simulink model "adarbha_HW9_sim_take2"  (Simulink 7.7)
settings: Solver=ode45  StartTime=0.0  StopTime=10.0  RelTol=1e-3
undefined symbols (not defined in the file): Area, Cd, density, Time, time_s, vel_m_s, Velocity_kph, weight_N
libraries: simulink x1
settings Model: Creator=Arjun  LastModifiedBy=Arjun

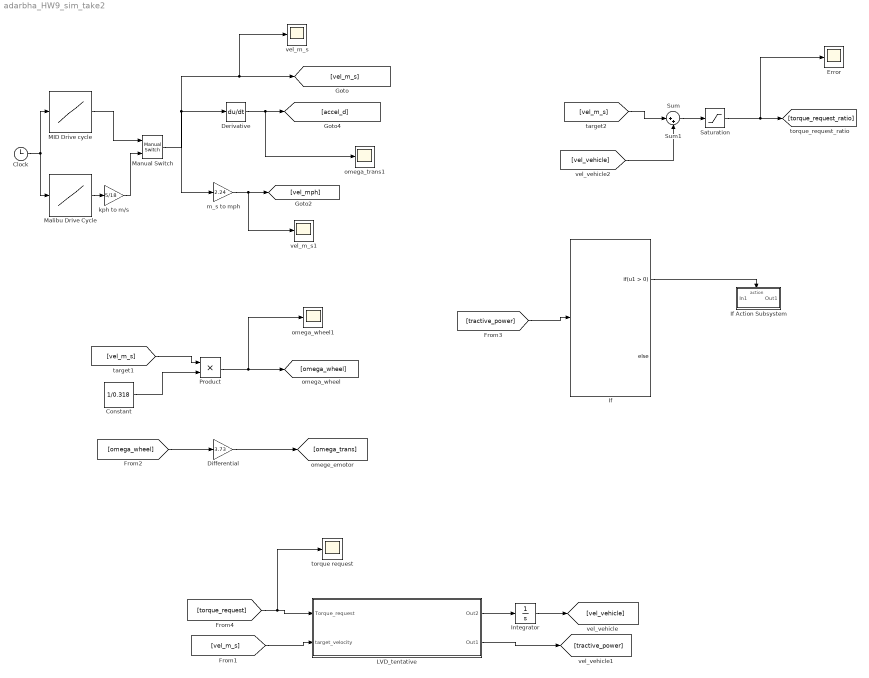
== system adarbha_HW9_sim_take2 ==
  Clock : Clock
      settings: Decimation=10
  Constant : Constant  Value=1/0.318
  Derivative : Derivative
  Differential : Gain  Gain=3.73
  Error : Scope
      settings: SaveName=ScopeData11
  If : If
  If Action Subsystem : Subsystem  TreatAsAtomicUnit=on
  Integrator : Integrator
  LVD_tentative : Subsystem
  MID Drive cycle : Lookup_n-D  NumberOfTableDimensions=1  BreakpointsForDimension1=time_s  Table=vel_m_s  RndMeth=Simplest  InputSameDT=on
  Malibu Drive Cycle : Lookup_n-D  NumberOfTableDimensions=1  BreakpointsForDimension1=Time  Table=Velocity_kph  RndMeth=Simplest  InputSameDT=on
  Manual Switch : simulink/Signal Routing/Manual Switch  SystemSampleTime=-1  sw=0  action=0  varsize=off
  Product : Product  RndMeth=Zero
  Saturation : Saturate  UpperLimit=1  LowerLimit=-1
  Sum : Sum  Inputs=|+-
  Sum1 : Sum  Inputs=|++
  kph to m/s : Gain  Gain=5/18
  m_s to mph : Gain  Gain=2.24
  omega_trans1 : Scope
      settings: YMin=0  YMax=40
  omega_wheel1 : Scope
      settings: SaveName=ScopeData3
  torque request : Scope
      settings: SaveName=ScopeData4
  vel_m_s : Scope
      settings: TimeRange=49.80784012298233  YMin=0  YMax=30
  vel_m_s1 : Scope
      settings: YMin=0  YMax=40  SaveName=ScopeData2
  wires:
  m_s to mph/1 -> [vel_mph], vel_m_s1/1
  Clock/1 -> MID Drive cycle/1, Malibu Drive Cycle/1
  MID Drive cycle/1 -> Manual Switch/1
  Manual Switch/1 -> m_s to mph/1, [vel_m_s], vel_m_s/1, Derivative/1
  Malibu Drive Cycle/1 -> kph to m/s/1
  kph to m/s/1 -> Manual Switch/2
  Derivative/1 -> [accel_d], omega_trans1/1
  [vel_m_s] -> Product/1
  Product/1 -> [omega_wheel], omega_wheel1/1
  Constant/1 -> Product/2
  [omega_wheel] -> Differential/1
  Differential/1 -> [omega_trans]
  [vel_m_s] -> LVD_tentative/2(target_velocity)
  [torque_request] -> LVD_tentative/1(Torque_request), torque request/1
  Integrator/1 -> [vel_vehicle]
  LVD_tentative/1(Out2) -> Integrator/1
  [vel_m_s] -> Sum/1
  [vel_vehicle] -> Sum/2
  Sum/1 -> Saturation/1
  Saturation/1 -> Error/1, [torque_request_ratio]
  LVD_tentative/2(Out1) -> [tractive_power]
  [tractive_power] -> If/1
  If/1 -> If Action Subsystem/Action

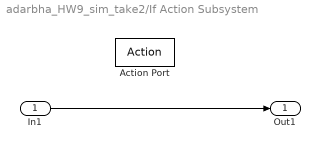
== system adarbha_HW9_sim_take2/If Action Subsystem ==
  In1 : Inport
  Action Port : ActionPort  ActionType=then
  Out1 : Outport
  wires:
  In1/1 -> Out1/1

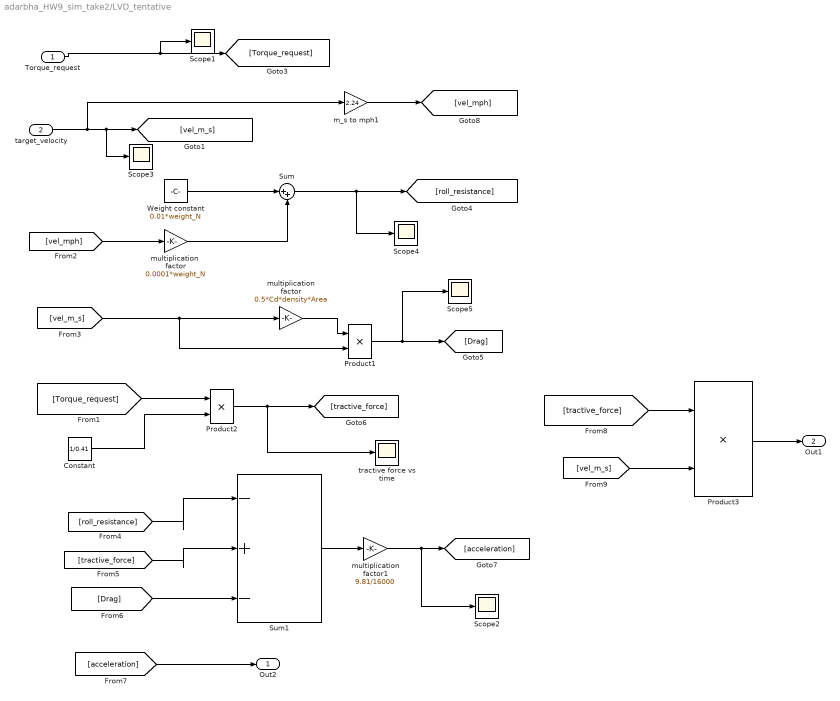
== system adarbha_HW9_sim_take2/LVD_tentative ==
  Torque_request : Inport
  target_velocity : Inport  Port=2
  Constant : Constant  Value=1/0.41
  Product1 : Product  RndMeth=Zero
  Product2 : Product  RndMeth=Zero
  Product3 : Product  RndMeth=Zero
  Scope{1..5} (5 alike) : Scope
      Scope1 settings: SaveName=ScopeData5
      Scope2 settings: SaveName=ScopeData6
      Scope3 settings: SaveName=ScopeData8
      Scope4 settings: SaveName=ScopeData9
      Scope5 settings: SaveName=ScopeData10
  Sum : Sum  Inputs=|++
  Sum1 : Sum  Inputs=|-+-
  Weight constant : Constant  Value=0.01*weight_N
  m_s to mph1 : Gain  Gain=2.24
  multiplication  factor : Gain  Gain=0.0001*weight_N
  multiplication factor : Gain  Gain=0.5*Cd*density*Area
  multiplication factor1 : Gain  Gain=9.81/16000
  tractive force vs time : Scope
      settings: SaveName=ScopeData13
  Out2 : Outport
  Out1 : Outport  Port=2
  wires:
  Weight constant/1 -> Sum/1
  multiplication  factor/1 -> Sum/2
  Sum/1 -> [roll_resistance], Scope4/1
  [vel_mph] -> multiplication  factor/1
  multiplication factor/1 -> Product1/1
  [vel_m_s] -> multiplication factor/1, Product1/2
  Product1/1 -> [Drag], Scope5/1
  [Torque_request] -> Product2/1
  Constant/1 -> Product2/2
  Product2/1 -> [tractive_force], tractive force vs time/1
  [roll_resistance] -> Sum1/1
  [tractive_force] -> Sum1/2
  [Drag] -> Sum1/3
  Sum1/1 -> multiplication factor1/1
  multiplication factor1/1 -> [acceleration], Scope2/1
  Torque_request/1 -> [Torque_request], Scope1/1
  target_velocity/1 -> m_s to mph1/1, [vel_m_s], Scope3/1
  m_s to mph1/1 -> [vel_mph]
  [acceleration] -> Out2/1
  [tractive_force] -> Product3/1
  [vel_m_s] -> Product3/2
  Product3/1 -> Out1/1
